simulink model "three_ph_imp_meas_dev"  (R2020b)
settings: Solver=FixedStepAuto  StartTime=0.0  StopTime=tStop  FixedStep=tStep  RelTol=1e-3
values from neighbouring files (symbols this model uses):
  amp = [0, amplitude]    [dq_new.m]    (also in dq_small.m = [0, 1]; dq_test.m)
  f_c = 50    [dq_new.m]    (also in dq_small.m; dq_test.m)
  freq = [f_meas f_meas]    [dq_new.m]    (also in dq_small.m = [f_p f_p]; dq_test.m = [freq_meas(1,i) freq_meas(1,i)]; test1.m = logspace(-2,4,20))
libraries: powerlib x9, powerlib_meascontrol x7
settings Model: Creator=kacper  LastModifiedBy=kacper

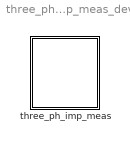
== system three_ph_imp_meas_dev ==
  three_ph_imp_meas : Subsystem

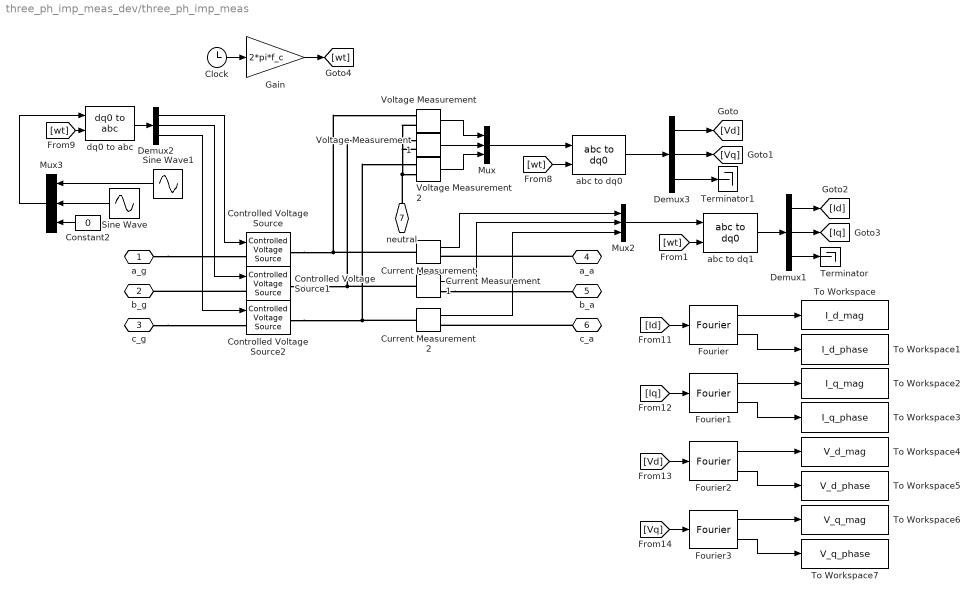
== system three_ph_imp_meas_dev/three_ph_imp_meas ==
  Clock : Clock
  Constant2 : Constant  Value=0
  Controlled Voltage Source : powerlib/Electrical Sources/Controlled Voltage Source  Initialize=on  Source_Type=AC  Amplitude=0  Phase=0  Frequency=0  Measurements=None
  Controlled Voltage Source1 : powerlib/Electrical Sources/Controlled Voltage Source  Initialize=on  Source_Type=AC  Amplitude=0  Phase=0  Frequency=0  Measurements=None
  Controlled Voltage Source2 : powerlib/Electrical Sources/Controlled Voltage Source  Initialize=on  Source_Type=AC  Amplitude=0  Phase=0  Frequency=0  Measurements=None
  Current Measurement : powerlib/Measurements/Current Measurement  PhasorSimulation=off  OutputType=Complex  PSBequivalent=0
  Current Measurement1 : powerlib/Measurements/Current Measurement  PhasorSimulation=off  OutputType=Complex  PSBequivalent=0
  Current Measurement2 : powerlib/Measurements/Current Measurement  PhasorSimulation=off  OutputType=Complex  PSBequivalent=0
  Demux1 : Demux  Outputs=3
  Demux2 : Demux  Outputs=3
  Demux3 : Demux  Outputs=3
  Fourier{,1..3} (4 alike) : powerlib_meascontrol/Measurements/Fourier  Freq=freq(1,1)  n=1  InInit=[0, 90]  Ts=0
  Gain : Gain  Gain=2*pi*f_c
  Mux : Mux  Inputs=3
  Mux2 : Mux  Inputs=3
  Mux3 : Mux  Inputs=3
  Sine Wave : Sin  Amplitude=amp(1,2)  Frequency=2*pi*freq(1,2)  SampleTime=0
  Sine Wave1 : Sin  Amplitude=amp(1,1)  Frequency=2*pi*freq(1,1)  SampleTime=0
  Terminator : Terminator
  Terminator1 : Terminator
  To Workspace : ToWorkspace  VariableName=I_d_mag  SampleTime=-1
  To Workspace1 : ToWorkspace  VariableName=I_d_phase  SampleTime=-1
  To Workspace2 : ToWorkspace  VariableName=I_q_mag  SampleTime=-1
  To Workspace3 : ToWorkspace  VariableName=I_q_phase  SampleTime=-1
  To Workspace4 : ToWorkspace  VariableName=V_d_mag  SampleTime=-1
  To Workspace5 : ToWorkspace  VariableName=V_d_phase  SampleTime=-1
  To Workspace6 : ToWorkspace  VariableName=V_q_mag  SampleTime=-1
  To Workspace7 : ToWorkspace  VariableName=V_q_phase  SampleTime=-1
  Voltage Measurement : powerlib/Measurements/Voltage Measurement  PhasorSimulation=off  OutputType=Complex  PSBequivalent=0
  Voltage Measurement1 : powerlib/Measurements/Voltage Measurement  PhasorSimulation=off  OutputType=Complex  PSBequivalent=0
  Voltage Measurement2 : powerlib/Measurements/Voltage Measurement  PhasorSimulation=off  OutputType=Complex  PSBequivalent=0
  abc to dq0 : powerlib_meascontrol/Transformations/abc to dq0  Alignment=90 degrees behind phase A axis
  abc to dq1 : powerlib_meascontrol/Transformations/abc to dq0  Alignment=90 degrees behind phase A axis
  dq0 to abc : powerlib_meascontrol/Transformations/dq0 to abc  Alignment=90 degrees behind phase A axis
  a_g : PMIOPort  Side=Left
  b_g : PMIOPort  Port=2  Side=Left
  c_g : PMIOPort  Port=3  Side=Left
  a_a : PMIOPort  Port=4  Side=Right
  b_a : PMIOPort  Port=5  Side=Right
  c_a : PMIOPort  Port=6  Side=Right
  neutral : PMIOPort  Port=7  Side=Left
  wires:
  [wt] -> abc to dq0/2
  Mux3/1 -> dq0 to abc/1
  Gain/1 -> [wt]
  Constant2/1 -> Mux3/3
  Demux1/3 -> Terminator/1
  Current Measurement2/1 -> Mux2/3
  Demux2/3 -> Controlled Voltage Source2/1
  [wt] -> dq0 to abc/2
  Demux3/1 -> [Vd]
  Fourier/1 -> To Workspace/1
  Voltage Measurement2/1 -> Mux/3
  Clock/1 -> Gain/1
  Demux3/2 -> [Vq]
  Sine Wave/1 -> Mux3/2
  Demux1/1 -> [Id]
  Voltage Measurement1/1 -> Mux/2
  dq0 to abc/1 -> Demux2/1
  Demux2/1 -> Controlled Voltage Source/1
  [Vq] -> Fourier3/1
  [Vd] -> Fourier2/1
  Fourier2/2 -> To Workspace5/1
  abc to dq1/1 -> Demux1/1
  Fourier3/1 -> To Workspace6/1
  Sine Wave1/1 -> Mux3/1
  Demux1/2 -> [Iq]
  Fourier1/2 -> To Workspace3/1
  [Iq] -> Fourier1/1
  Mux2/1 -> abc to dq1/1
  Fourier3/2 -> To Workspace7/1
  Current Measurement1/1 -> Mux2/2
  [Id] -> Fourier/1
  abc to dq0/1 -> Demux3/1
  Demux3/3 -> Terminator1/1
  Mux/1 -> abc to dq0/1
  Fourier/2 -> To Workspace1/1
  Demux2/2 -> Controlled Voltage Source1/1
  Current Measurement/1 -> Mux2/1
  Fourier1/1 -> To Workspace2/1
  [wt] -> abc to dq1/2
  Voltage Measurement/1 -> Mux/1
  Fourier2/1 -> To Workspace4/1
  connections:
  a_g/RConn1 -- Controlled Voltage Source/LConn1
  c_g/RConn1 -- Controlled Voltage Source2/LConn1
  Current Measurement1/LConn1 -- Controlled Voltage Source1/RConn1 -- Voltage Measurement1/LConn1
  a_a/RConn1 -- Current Measurement/RConn1
  Controlled Voltage Source1/LConn1 -- b_g/RConn1
  Current Measurement1/RConn1 -- b_a/RConn1
  Current Measurement2/LConn1 -- Controlled Voltage Source2/RConn1 -- Voltage Measurement2/LConn1
  Current Measurement/LConn1 -- Controlled Voltage Source/RConn1 -- Voltage Measurement/LConn1
  Voltage Measurement/LConn2 -- Voltage Measurement1/LConn2 -- neutral/RConn1 -- Voltage Measurement2/LConn2
  c_a/RConn1 -- Current Measurement2/RConn1
